simulink model "PV_buck_boost_mppt"  (Simulink 7.1)
settings: Solver=ode45  StartTime=0.0  StopTime=7  RelTol=1e-3
undefined symbols (not defined in the file or in its folder): DiscIntNeverNeededParam
libraries: powerlib x12, simulink x1
settings Model: Creator=jagan  LastModifiedBy=jagan

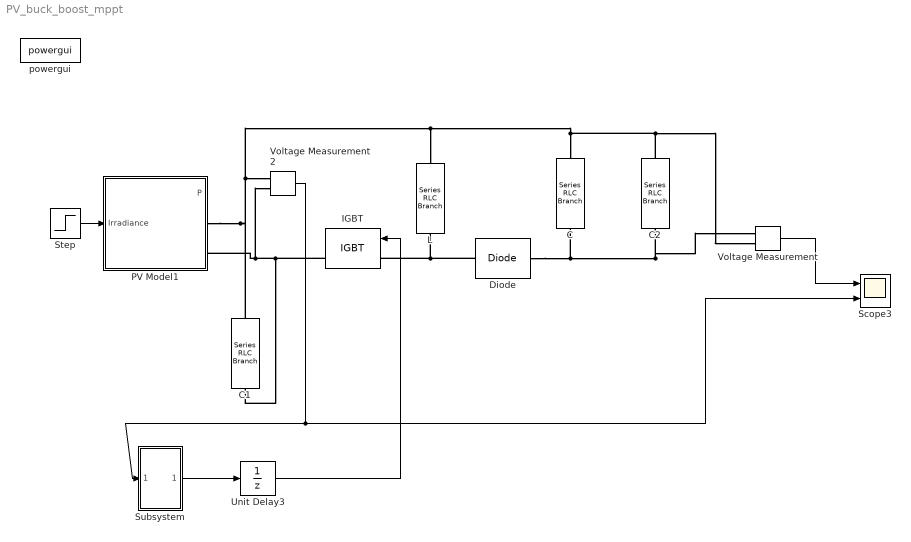
== system PV_buck_boost_mppt ==
  C : powerlib/Elements/Series RLC Branch  Orientation=up  DialogController=POWERSYS.PowerSysDialog  PhysicalDomain=powersysdomain  SubClassName=unknown  LeftPortType=p1  RightPortType=p1  LConnTagsString=__new0  RConnTagsString=__new0  BranchType=C  Resistance=1  Inductance=1e-3  SetiL0=off  InitialCurrent=0  Capacitance=2300e-6  Setx0=off  InitialVoltage=0  Measurements=None
  C1 : powerlib/Elements/Series RLC Branch  Orientation=up  DialogController=POWERSYS.PowerSysDialog  PhysicalDomain=powersysdomain  SubClassName=unknown  LeftPortType=p1  RightPortType=p1  LConnTagsString=__new0  RConnTagsString=__new0  BranchType=C  Resistance=1  Inductance=1e-3  SetiL0=off  InitialCurrent=0  Capacitance=2300e-6  Setx0=off  InitialVoltage=0  Measurements=None
  C2 : powerlib/Elements/Series RLC Branch  Orientation=up  DialogController=POWERSYS.PowerSysDialog  PhysicalDomain=powersysdomain  SubClassName=unknown  LeftPortType=p1  RightPortType=p1  LConnTagsString=__new0  RConnTagsString=__new0  BranchType=R  Resistance=10  Inductance=1e-3  SetiL0=off  InitialCurrent=0  Capacitance=2300e-6  Setx0=off  InitialVoltage=0  Measurements=None
  Diode : powerlib/Power Electronics/Diode  DialogController=POWERSYS.PowerSysDialog  SystemSampleTime=-1  Ron=0.001  Lon=0  Vf=0.8  IC=0  UseSnubber=off  Rs=500  Cs=250e-9  Measurements=off
  IGBT : powerlib/Power Electronics/IGBT  Orientation=left  DialogController=POWERSYS.PowerSysDialog  SystemSampleTime=-1  Ron=0.001  Lon=0  Vf=1  Tf=1e-6  Tt=2e-6  IC=0  Rs=1e5  Cs=inf  Measurements=on
  L : powerlib/Elements/Series RLC Branch  Orientation=up  DialogController=POWERSYS.PowerSysDialog  PhysicalDomain=powersysdomain  SubClassName=unknown  LeftPortType=p1  RightPortType=p1  LConnTagsString=__new0  RConnTagsString=__new0  BranchType=L  Resistance=1  Inductance=50e-3  SetiL0=off  InitialCurrent=0  Capacitance=1e-6  Setx0=off  InitialVoltage=0  Measurements=None
  PV Model1 : Subsystem  mask{Isc=8.79, Voc=44.97, Im=8.16, Vm=35.30, ns=1}
      mask prompts: Isc "Short-Circuit Current"; Voc "Open-Circuit Voltage"; Im "Current at Pmax"; Vm "Voltage at Pmax"; ns "Number of Modules connected in series"
      mask init:
      | % calculation of PV module parameters
      | % limitation: constant temperature
      | Ns = round(Voc/0.61); % default number of cells in series
      | Vt = 26e-3; % thermal voltage
      | G = Isc/1000; % irradiation to short-circuit current gain
      | Vmpc = Vm/Ns; % cell voltage at rated Pmax
      | Vocc = Voc/Ns; % cell open-circuit voltage
      | Rmpp = Vmpc/Im; % cell load resistance at Pmax
      | %
      | Rp = 100*Vocc/Isc; % initial value for Rp
      | Vdm = Vocc; % initial value for Vdm
      | %
      | % iterative solution for model parameters: Io, Rs, Rp
      | for i=1:10
      | %
      |  Idm = Isc - Im - Vdm/Rp; % pn-junction (diode) current at MPP
      |  Io = (Isc-Vocc/Rp)/(exp(Vocc/Vt)-1); % pn-junction reverse saturation current
      |  Vdm = Vt*log(Idm/Io+1); % pn-junction (diode) voltage at MPP
      |  Rs = (Vdm-Vmpc)/Im; % cell series resistance
      |  Rd = (Rmpp - Rs)*Rp/(Rp-Rmpp+Rs); % diode incremental resistance at MPP
      |  Idm = Vt/Rd; % diode current at MPP based on incremental resistance
      |  Rp = Vdm/(Isc-Im-Idm); % cell parallel resistance
      | %
      | end
      | %
  Scope3 : Scope  NumInputPorts=2
      settings: TimeRange=0.04  YMin=49.3~35.2  YMax=49.95~35.8  SaveName=ScopeData7  SampleInput=on
  Step : Step  Time=2  Before=1000  After=900  SampleTime=5e-5
  Subsystem : Subsystem
  Unit Delay3 : UnitDelay  SampleTime=-1
  Voltage Measurement : powerlib/Measurements/Voltage Measurement  DialogController=POWERSYS.PowerSysDialog  SystemSampleTime=-1  PhasorSimulation=off  OutputType=Complex  PSBequivalent=0
  Voltage Measurement2 : powerlib/Measurements/Voltage Measurement  DialogController=POWERSYS.PowerSysDialog  SystemSampleTime=-1  PhasorSimulation=off  OutputType=Complex  PSBequivalent=0
  powergui : powerlib/powergui  SystemSampleTime=-1  SimulationMode=Discrete  SampleTime=50e-6  frequency=60  SPID=off  SwTol=0  Interpol=off  x0status=blocks  echomessages=off  HookPort=off  FunctionMessages=off  EnableUseOfTLC=off  RestoreLinks=warning  frequencyindice=0  Frange=[0:2:500]  Ylog=off  Xlog=on  ShowGrid=off  save=off  variable=ZData  ZoomFFT=on  StartTime=0.0  cycles=1  DisplayStyle=1  fundamental=60  FreqAxis=off  MaxFrequency=1000  frequencyindicesteady=1  RmsSteady=1  display=off  Ts=0  methode=off
  wires:
  Step/1 -> PV Model1/1(Irradiance)
  Voltage Measurement2/1 -> Subsystem/1(Vdc), Scope3/2
  Subsystem/1(Out2) -> Unit Delay3/1
  Unit Delay3/1 -> IGBT/1
  Voltage Measurement/1 -> Scope3/1
  connections:
  Diode/LConn1 -- L/LConn1 -- IGBT/LConn1
  PV Model1/RConn1 -- C1/RConn1 -- Voltage Measurement2/LConn1 -- L/RConn1 -- C/RConn1 -- C2/RConn1 -- Voltage Measurement/LConn2
  Diode/RConn1 -- C/LConn1 -- C2/LConn1 -- Voltage Measurement/LConn1
  IGBT/RConn1 -- PV Model1/RConn2 -- Voltage Measurement2/LConn2 -- C1/LConn1

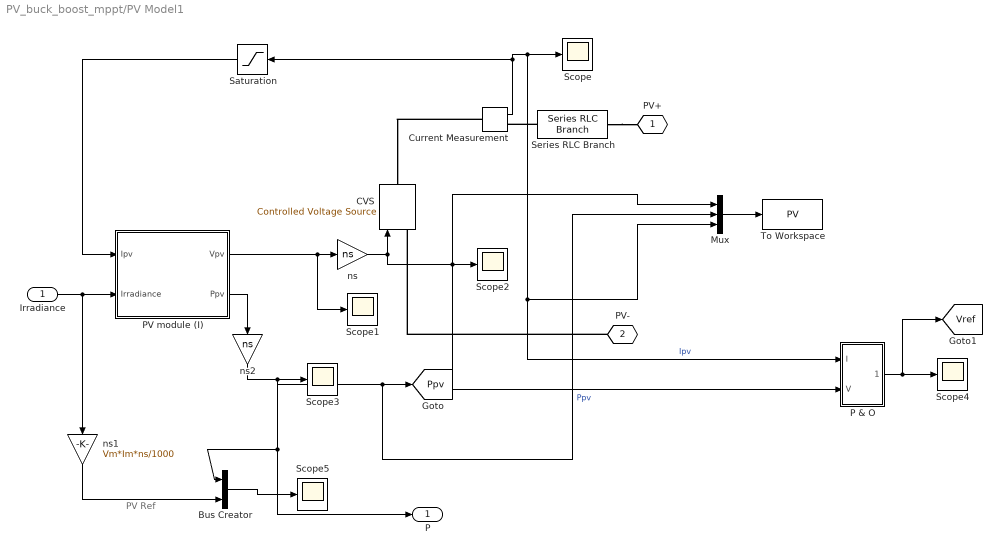
== system PV_buck_boost_mppt/PV Model1 ==
  note: PV Ref
  Irradiance : Inport  OutDataType=sfix(16)  OutScaling=2^0
  Bus Creator : BusCreator  Inputs=2
  CVS : powerlib/Electrical Sources/Controlled Voltage Source  Orientation=up  DialogController=POWERSYS.PowerSysDialog  SystemSampleTime=-1  Initialize=on  Source_Type=DC  Amplitude=0  Phase=0  Frequency=0  Measurements=None
  Current Measurement : powerlib/Measurements/Current Measurement  DialogController=POWERSYS.PowerSysDialog  SystemSampleTime=-1  PhasorSimulation=off  OutputType=Complex  PSBequivalent=0
  Mux : Mux  Inputs=3
  P & O : Subsystem
  PV module (I) : Subsystem
  Saturation : Saturate  Orientation=left  UpperLimit=inf  LowerLimit=0
  Scope{,1..5} (6 alike) : Scope
      Scope settings: YMin=-0.00726198  YMax=-0.00726198
      Scope1 settings: SaveName=ScopeData2
      Scope2 settings: YMin=805  YMax=809.5  SaveName=ScopeData3
      Scope3 settings: YMin=287.7  YMax=288.05  SaveName=ScopeData4
      Scope4 settings: YMin=35.258  YMax=35.2655  SaveName=ScopeData28
      Scope5 settings: YMin=257.5  YMax=290  SaveName=ScopeData42
  Series RLC Branch : powerlib/Elements/Series RLC Branch  DialogController=POWERSYS.PowerSysDialog  PhysicalDomain=powersysdomain  SubClassName=unknown  LeftPortType=p1  RightPortType=p1  LConnTagsString=__new0  RConnTagsString=__new0  BranchType=R  Resistance=0.00001  Inductance=1e-3  SetiL0=off  InitialCurrent=0  Capacitance=1e-6  Setx0=off  InitialVoltage=0  Measurements=None
  To Workspace : ToWorkspace  VariableName=PV  SampleTime=-1  SaveFormat=Structure With Time
  ns : Gain  Gain=ns  ParameterDataType=sfix(16)  ParameterScaling=2^0  OutDataType=sfix(16)  OutScaling=2^0
  ns1 : Gain  Orientation=down  Gain=Vm*Im*ns/1000  ParameterDataType=sfix(16)  ParameterScaling=2^0  OutDataType=sfix(16)  OutScaling=2^0
  ns2 : Gain  Orientation=down  Gain=ns  ParameterDataType=sfix(16)  ParameterScaling=2^0  OutDataType=sfix(16)  OutScaling=2^0
  PV+ : PMIOPort  Tag=PMCPort  Orientation=left  Port=1  Side=Right
  PV- : PMIOPort  Tag=PMCPort  Orientation=left  Port=2  Side=Right
  P : Outport  OutDataType=sfix(16)  OutScaling=2^0
  tag scope: Ppv=global, Vref=global
  wires:
  ns2/1 -> Scope3/1, [Ppv], Mux/2, Bus Creator/1, P/1  "Ppv"
  ns/1 -> CVS/1, Scope2/1, Mux/1, P & O/2(V)
  PV module (I)/2(Ppv) -> ns2/1
  Irradiance/1 -> PV module (I)/2(Irradiance), ns1/1
  Current Measurement/1 -> Scope/1, Mux/3, P & O/1(I), Saturation/1  "Ipv"
  PV module (I)/1(Vpv) -> Scope1/1, ns/1
  Mux/1 -> To Workspace/1
  P & O/1(Vref) -> Scope4/1, [Vref]
  ns1/1 -> Bus Creator/2
  Bus Creator/1 -> Scope5/1
  Saturation/1 -> PV module (I)/1(Ipv)
  connections:
  Series RLC Branch/LConn1 -- Current Measurement/RConn1
  Current Measurement/LConn1 -- CVS/RConn1
  PV-/RConn1 -- CVS/LConn1
  Series RLC Branch/RConn1 -- PV+/RConn1

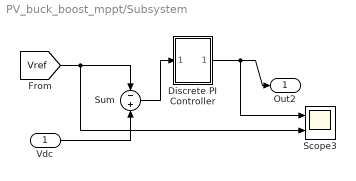
== system PV_buck_boost_mppt/Subsystem ==
  Vdc : Inport  OutDataType=sfix(16)  OutScaling=2^0
  Discrete PI Controller : Subsystem  AncestorBlock=|  DialogController=POWERSYS.PowerSysDialog  mask(Discrete PI Controller){Kp=1, Ki=85, Par_Limits=[1 0], Init=0, Ts=20e-6}
      | powerlib_extras/Discrete 
      | Control Blocks/Discrete
      | PI Controller
      mask prompts: Kp "Proportional gain (Kp):"; Ki "Integral gain (Ki):"; Par_Limits "Output limits: [ Upper   Lower ]"; Init "Output initial value:"; Ts "Sample time:"
      mask help: This block implements a discrete PI controller.
      mask init:
      | UpperLimit=Par_Limits(1);
      | LowerLimit=Par_Limits(2);
      | power_initmask();
      mask Help: This block is part of a subset of blocks in the Extras library that does not have documentation associated with it, other than the block mask description.
      mask Display: disp('PI');
  Scope3 : Scope  NumInputPorts=2
      settings: TimeRange=0.04  YMin=0.75~35.258  YMax=1~35.2655  SaveName=ScopeData5  SampleInput=on
  Sum : Sum  Inputs=-+  OutDataType=sfix(16)  OutScaling=2^0  SaturateOnIntegerOverflow=on  InputSameDT=on  OutDataTypeStr=Inherit: Same as first input
  Out2 : Outport
  wires:
  Sum/1 -> Discrete PI Controller/1(Error)
  Vdc/1 -> Sum/2
  [Vref] -> Sum/1, Scope3/2
  Discrete PI Controller/1(Out) -> Out2/1, Scope3/1

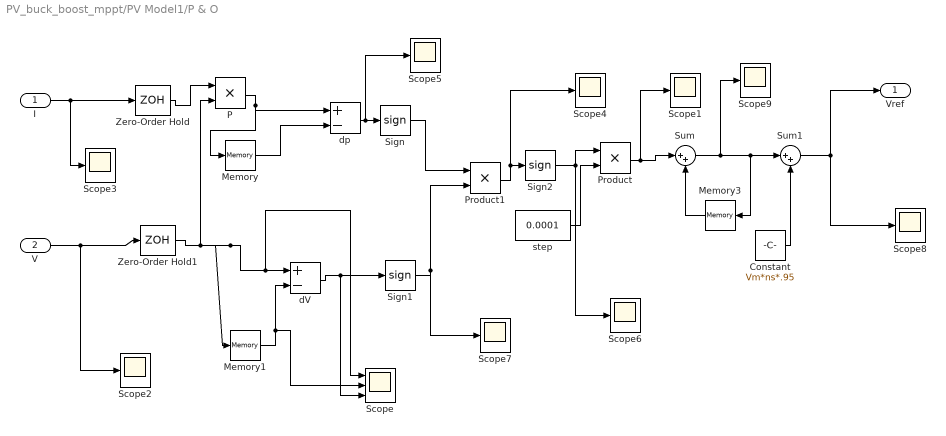
== system PV_buck_boost_mppt/PV Model1/P & O ==
  I : Inport  OutDataType=sfix(16)  OutScaling=2^0
  V : Inport  Port=2  OutDataType=sfix(16)  OutScaling=2^0
  Constant : Constant  Value=Vm*ns*.95  OutDataType=sfix(16)  OutScaling=2^0
  Memory : Memory  InheritSampleTime=on
  Memory1 : Memory  InheritSampleTime=on
  Memory3 : Memory  Orientation=left  InheritSampleTime=on
  P : Product  OutDataType=sfix(16)  OutScaling=2^0  RndMeth=Zero
  Product : Product  OutDataType=sfix(16)  OutScaling=2^0  RndMeth=Zero
  Product1 : Product  OutDataType=sfix(16)  OutScaling=2^0  RndMeth=Zero
  Scope : Scope  NumInputPorts=3
      settings: YMin=29.1717~29.1717~1e-006  YMax=32.2424~32.2424~1.7e-005
  Scope{1..9} (9 alike) : Scope
      Scope1 settings: YMin=-0.0005  YMax=0.0005  SaveName=ScopeData34
      Scope2 settings: YMin=-11  YMax=10  SaveName=ScopeData35
      Scope3 settings: YMin=-11  YMax=10  SaveName=ScopeData36
      Scope4 settings: YMin=-11  YMax=10  SaveName=ScopeData37
      Scope5 settings: YMin=-11  YMax=10
      Scope6 settings: YMin=-11  YMax=10  SaveName=ScopeData38
      Scope7 settings: YMin=-11  YMax=10  SaveName=ScopeData39
      Scope8 settings: YMin=657.75  YMax=658.275  SaveName=ScopeData40
      Scope9 settings: YMin=-7.5  YMax=2.5  SaveName=ScopeData41
  Sign : Signum
  Sign1 : Signum
  Sign2 : Signum
  Sum : Sum  Inputs=|++  OutDataType=sfix(16)  OutScaling=2^0
  Sum1 : Sum  Inputs=|++  OutDataType=sfix(16)  OutScaling=2^0
  Zero-Order Hold : ZeroOrderHold  SampleTime=0.0002
  Zero-Order Hold1 : ZeroOrderHold  SampleTime=0.0002
  dV : Sum  Inputs=+-  OutDataType=sfix(16)  OutScaling=2^-10
  dp : Sum  Inputs=+-  OutDataType=sfix(16)  OutScaling=2^-10
  step : Constant  Value=0.0001  OutDataType=sfix(16)  OutScaling=2^0
  Vref : Outport  OutDataType=sfix(16)  OutScaling=2^0
  wires:
  Memory1/1 -> dV/2, Scope/2
  Memory/1 -> dp/2
  V/1 -> Zero-Order Hold1/1, Scope2/1
  dV/1 -> Sign1/1, Scope/3
  step/1 -> Product/2
  Product/1 -> Sum/1, Scope1/1
  Sign/1 -> Product1/1
  Sign1/1 -> Product1/2, Scope7/1
  Product1/1 -> Sign2/1, Scope4/1
  I/1 -> Zero-Order Hold/1, Scope3/1
  Zero-Order Hold1/1 -> P/2, Memory1/1, dV/1, Scope/1
  Zero-Order Hold/1 -> P/1
  P/1 -> Memory/1, dp/1
  dp/1 -> Sign/1, Scope5/1
  Sign2/1 -> Product/1, Scope6/1
  Sum/1 -> Memory3/1, Sum1/1, Scope9/1
  Memory3/1 -> Sum/2
  Sum1/1 -> Vref/1, Scope8/1
  Constant/1 -> Sum1/2

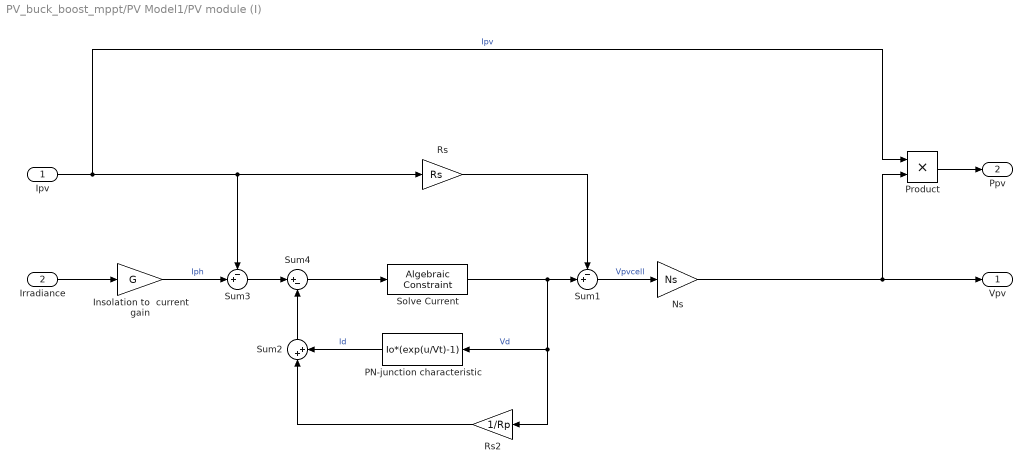
== system PV_buck_boost_mppt/PV Model1/PV module (I) ==
  Ipv : Inport  OutDataType=sfix(16)  OutScaling=2^0
  Irradiance : Inport  Port=2  OutDataType=sfix(16)  OutScaling=2^0
  Insolation to  current gain : Gain  Gain=G  ParameterDataType=sfix(16)  ParameterScaling=2^0  OutDataType=sfix(16)  OutScaling=2^0
  Ns : Gain  Gain=Ns  ParameterDataType=sfix(16)  ParameterScaling=2^0  OutDataType=sfix(16)  OutScaling=2^0
  PN-junction characteristic : Fcn  Orientation=left  Expr=Io*(exp(u/Vt)-1)
  Product : Product  OutDataType=sfix(16)  OutScaling=2^0  RndMeth=Zero
  Rs : Gain  Gain=Rs  ParameterDataType=sfix(16)  ParameterScaling=2^0  OutDataType=sfix(16)  OutScaling=2^0
  Rs2 : Gain  Orientation=left  Gain=1/Rp  ParameterDataType=sfix(16)  ParameterScaling=2^0  OutDataType=sfix(16)  OutScaling=2^0
  Solve Current : simulink/Math Operations/Algebraic Constraint  SystemSampleTime=-1  z0=1.99
  Sum1 : Sum  Inputs=-+|  OutDataType=sfix(16)  OutScaling=2^0
  Sum2 : Sum  Orientation=up  Inputs=|++  OutDataType=sfix(16)  OutScaling=2^0
  Sum3 : Sum  Inputs=-+|  OutDataType=sfix(16)  OutScaling=2^0
  Sum4 : Sum  Inputs=|+-  OutDataType=sfix(16)  OutScaling=2^0
  Vpv : Outport  OutDataType=sfix(16)  OutScaling=2^0
  Ppv : Outport  Port=2  OutDataType=sfix(16)  OutScaling=2^0
  wires:
  PN-junction characteristic/1 -> Sum2/2  "Id"
  Sum3/1 -> Sum4/1
  Ns/1 -> Product/2, Vpv/1
  Rs/1 -> Sum1/1
  Sum1/1 -> Ns/1  "Vpvcell"
  Solve Current/1 -> Sum1/2, PN-junction characteristic/1, Rs2/1  "Vd"
  Sum4/1 -> Solve Current/1
  Product/1 -> Ppv/1
  Ipv/1 -> Rs/1, Sum3/1, Product/1  "Ipv"
  Insolation to  current gain/1 -> Sum3/2  "Iph"
  Irradiance/1 -> Insolation to  current gain/1
  Rs2/1 -> Sum2/1
  Sum2/1 -> Sum4/2

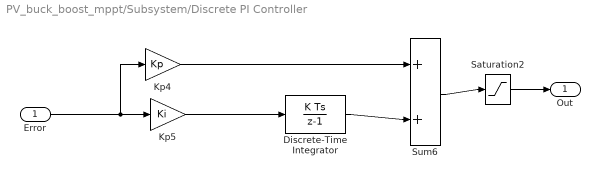
== system PV_buck_boost_mppt/Subsystem/Discrete PI Controller ==
  Error : Inport  OutDataType=sfix(16)  OutScaling=2^0
  Discrete-Time Integrator : DiscreteIntegrator  InitialCondition=Init  SampleTime=Ts  OutDataType=sfix(16)  OutScaling=2^0  LimitOutput=on  UpperSaturationLimit=UpperLimit  LowerSaturationLimit=LowerLimit  ICPrevOutput=DiscIntNeverNeededParam  ICPrevScaledInput=DiscIntNeverNeededParam
  Kp4 : Gain  Gain=Kp  ParameterDataType=sfix(16)  ParameterScaling=2^0  OutDataType=sfix(16)  OutScaling=2^0  SaturateOnIntegerOverflow=on  OutDataTypeStr=Inherit: Same as input  ParamDataTypeStr=Inherit: Same as input
  Kp5 : Gain  Gain=Ki  ParameterDataType=sfix(16)  ParameterScaling=2^0  OutDataType=sfix(16)  OutScaling=2^0  SaturateOnIntegerOverflow=on  OutDataTypeStr=Inherit: Same as input  ParamDataTypeStr=Inherit: Same as input
  Saturation2 : Saturate  UpperLimit=UpperLimit  LowerLimit=LowerLimit
  Sum6 : Sum  OutDataType=sfix(16)  OutScaling=2^0  SaturateOnIntegerOverflow=on  InputSameDT=on  OutDataTypeStr=Inherit: Same as first input
  Out : Outport  OutDataType=sfix(16)  OutScaling=2^0  InitialOutput=0
  wires:
  Saturation2/1 -> Out/1
  Discrete-Time Integrator/1 -> Sum6/2
  Kp4/1 -> Sum6/1
  Kp5/1 -> Discrete-Time Integrator/1
  Sum6/1 -> Saturation2/1
  Error/1 -> Kp5/1, Kp4/1
